simulink model "bilinear"  (R2020a)
settings: Solver=VariableStepAuto  StartTime=0.0  StopTime=10.0  RelTol=1e-3
settings Model: Creator=Jake  LastModifiedBy=Jake

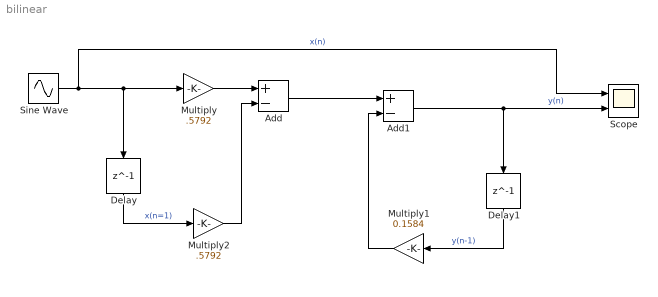
== system bilinear ==
  Add : Sum  Inputs=+-
  Add1 : Sum  Inputs=+-
  Delay : Delay  DelayLength=1
  Delay1 : Delay  DelayLength=1
  Multiply : Gain  Gain=.5792
  Multiply1 : Gain  Gain=0.1584
  Multiply2 : Gain  Gain=.5792
  Scope : Scope  NumInputPorts=2
  Sine Wave : Sin  Frequency=10*6.28  SampleTime=0
  wires:
  Sine Wave/1 -> Scope/1, Multiply/1, Delay/1  "x(n)"
  Multiply/1 -> Add/1
  Delay1/1 -> Multiply1/1  "y(n-1)"
  Add/1 -> Add1/1
  Multiply1/1 -> Add1/2
  Add1/1 -> Delay1/1, Scope/2  "y(n)"
  Delay/1 -> Multiply2/1  "x(n=1)"
  Multiply2/1 -> Add/2
